simulink model "sim_linear_control_pos_v1"  (R2018a)
settings: Solver=ode3  StartTime=0.0  StopTime=t(end)  FixedStep=dt  RelTol=1e-3
values from neighbouring files (symbols this model uses):
  A = [-(Cf+Cr)/(m*Vx)  -(a*Cf-b*Cr)/(m*Vx)-Vx ... (first row only)    [lin_control_pos_v1.m]    (also in lin_control_y.m)
  B = [Cf/m; a*Cf/Iz]    [lin_control_pos_v1.m]    (also in lin_control_y.m)
  C = Col(3,:)    [lin_control_pos_v1.m]    (also in lin_control_y.m)
  CA = C*Aol    [lin_control_pos_v1.m]    (also in lin_control_y.m)
  invCB = pinv(C*Bol)    [lin_control_pos_v1.m]    (also in lin_control_y.m)
  K_ay = 8    [lin_control_pos_v1.m]    (also in lin_control_y.m = 4)
  K_chi = 2    [lin_control_pos_v1.m]
  K_Vy = 4    [lin_control_pos_v1.m]
  rho = 1/R    (= 0.05)    [lin_control_pos_v1.m]    (also in lin_control_y.m)
  Vx = 10/3.6    (= 2.77777777778)    [lin_control_pos_v1.m]    (also in lin_control_y.m)
  w = 10    [lin_control_pos_v1.m]    (also in lin_control_y.m)
settings Model: Creator=E183308  LastModifiedBy=E183308

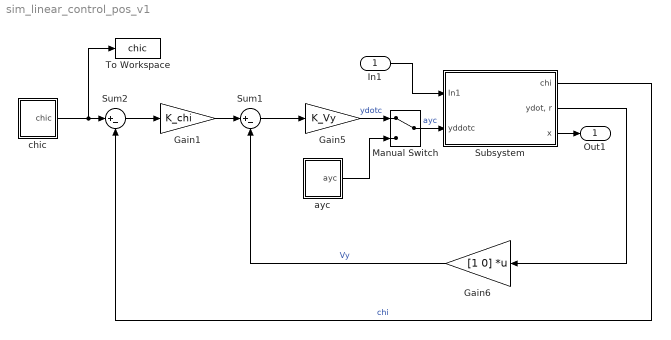
== system sim_linear_control_pos_v1 ==
  In1 : Inport
  Gain1 : Gain  Gain=K_chi
  Gain5 : Gain  Gain=K_Vy
  Gain6 : Gain  Gain=[1 0]  Multiplication=Matrix(K*u)
  Manual Switch : ManualSwitch
  Subsystem : Subsystem
  Sum1 : Sum  Inputs=|+-
  Sum2 : Sum  Inputs=|+-
  To Workspace : ToWorkspace  VariableName=chic  SampleTime=-1
  ayc : Subsystem
  chic : Subsystem
  Out1 : Outport
  wires:
  Gain5/1 -> Manual Switch/1  "ydotc"
  Sum1/1 -> Gain5/1
  Gain6/1 -> Sum1/2  "Vy"
  In1/1 -> Subsystem/1(In1)
  Manual Switch/1 -> Subsystem/2(yddotc)  "ayc"
  Subsystem/2("ydot, r") -> Gain6/1
  Subsystem/3(x) -> Out1/1
  Gain1/1 -> Sum1/1
  ayc/1(ayc) -> Manual Switch/2
  Subsystem/1(chi) -> Sum2/2  "chi"
  Sum2/1 -> Gain1/1
  chic/1(chic) -> To Workspace/1, Sum2/1

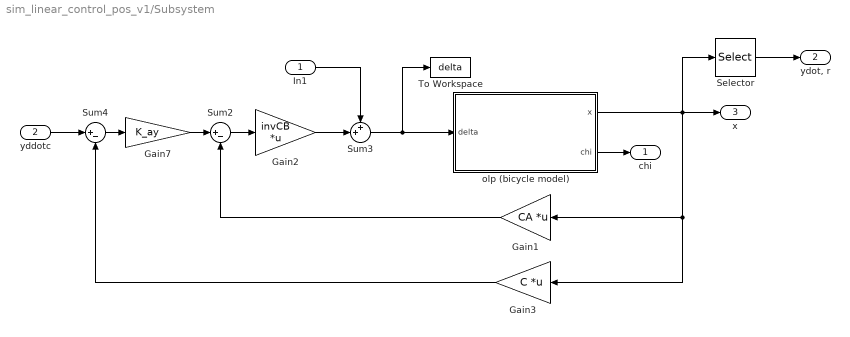
== system sim_linear_control_pos_v1/Subsystem ==
  In1 : Inport
  yddotc : Inport  Port=2
  Gain1 : Gain  Gain=CA  Multiplication=Matrix(K*u)
  Gain2 : Gain  Gain=invCB  Multiplication=Matrix(K*u)
  Gain3 : Gain  Gain=C  Multiplication=Matrix(K*u)
  Gain7 : Gain  Gain=K_ay
  Selector : Selector  InputPortWidth=5  IndexOptions=Index vector (dialog)  Indices=[1 2]  OutputSizes=1
  Sum2 : Sum  Inputs=|+-
  Sum3 : Sum  Inputs=++|
  Sum4 : Sum  Inputs=|+-
  To Workspace : ToWorkspace  VariableName=delta  SampleTime=-1
  olp (bicycle model) : Subsystem
  chi : Outport
  "ydot, r" : Outport  Port=2
  x : Outport  Port=3
  wires:
  yddotc/1 -> Sum4/1
  Gain3/1 -> Sum4/2
  Sum2/1 -> Gain2/1
  Sum4/1 -> Gain7/1
  Gain1/1 -> Sum2/2
  Gain7/1 -> Sum2/1
  olp (bicycle model)/1(x) -> Gain3/1, Gain1/1, x/1, Selector/1
  Selector/1 -> "ydot, r"/1
  Gain2/1 -> Sum3/2
  Sum3/1 -> To Workspace/1, olp (bicycle model)/1(delta)
  In1/1 -> Sum3/1
  olp (bicycle model)/2(chi) -> chi/1

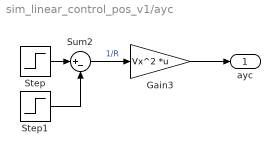
== system sim_linear_control_pos_v1/ayc ==
  Gain3 : Gain  Gain=Vx^2  Multiplication=Matrix(K*u)
  Step : Step  After=rho  SampleTime=0
  Step1 : Step  Time=5  After=rho  SampleTime=0
  Sum2 : Sum  Inputs=|+-
  ayc : Outport
  wires:
  Step1/1 -> Sum2/2
  Step/1 -> Sum2/1
  Sum2/1 -> Gain3/1  "1/R"
  Gain3/1 -> ayc/1

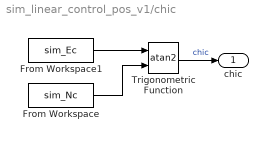
== system sim_linear_control_pos_v1/chic ==
  From Workspace : FromWorkspace  VariableName=sim_Nc  SampleTime=0
  From Workspace1 : FromWorkspace  VariableName=sim_Ec  SampleTime=0
  Trigonometric Function : Trigonometry  Operator=atan2
  chic : Outport
  wires:
  From Workspace1/1 -> Trigonometric Function/1
  From Workspace/1 -> Trigonometric Function/2
  Trigonometric Function/1 -> chic/1  "chic"

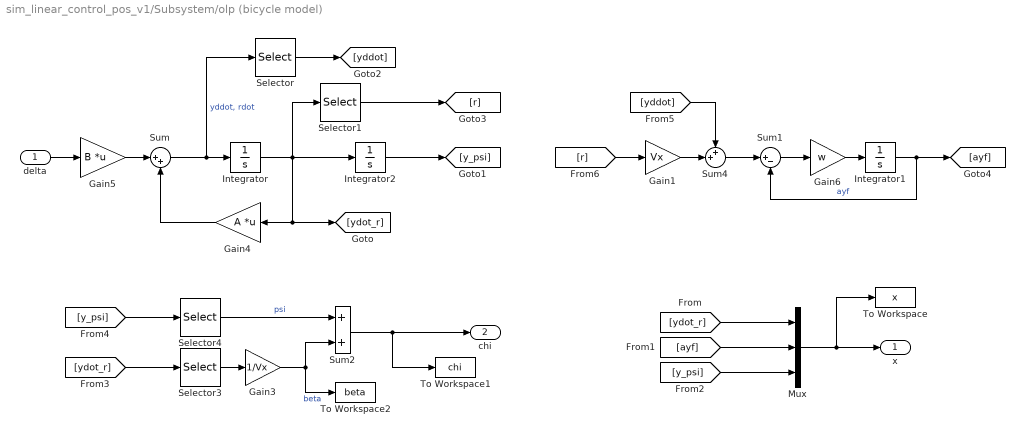
== system sim_linear_control_pos_v1/Subsystem/olp (bicycle model) ==
  delta : Inport
  Gain1 : Gain  Gain=Vx
  Gain3 : Gain  Gain=1/Vx
  Gain4 : Gain  Gain=A  Multiplication=Matrix(K*u)
  Gain5 : Gain  Gain=B  Multiplication=Matrix(K*u)
  Gain6 : Gain  Gain=w
  Integrator : Integrator  InitialCondition=[0;0]
  Integrator1 : Integrator
  Integrator2 : Integrator  InitialCondition=[0;0]
  Mux : Mux  Inputs=3
  Selector : Selector  InputPortWidth=2  IndexOptions=Index vector (dialog)  Indices=1  OutputSizes=1
  Selector1 : Selector  InputPortWidth=2  IndexOptions=Index vector (dialog)  Indices=2  OutputSizes=1
  Selector3 : Selector  InputPortWidth=2  IndexOptions=Index vector (dialog)  Indices=1  OutputSizes=1
  Selector4 : Selector  InputPortWidth=2  IndexOptions=Index vector (dialog)  Indices=2  OutputSizes=1
  Sum : Sum  Inputs=|++
  Sum1 : Sum  Inputs=|+-
  Sum2 : Sum
  Sum4 : Sum  Inputs=++|
  To Workspace : ToWorkspace  VariableName=x  SampleTime=-1
  To Workspace1 : ToWorkspace  VariableName=chi  SampleTime=-1
  To Workspace2 : ToWorkspace  VariableName=beta  SampleTime=-1
  x : Outport
  chi : Outport  Port=2
  wires:
  Integrator/1 -> Selector1/1, Integrator2/1, [ydot_r], Gain4/1
  delta/1 -> Gain5/1
  Gain5/1 -> Sum/1
  Gain4/1 -> Sum/2
  Gain6/1 -> Integrator1/1
  Sum1/1 -> Gain6/1
  Mux/1 -> x/1, To Workspace/1
  Integrator1/1 -> [ayf], Sum1/2  "ayf"
  Sum/1 -> Selector/1, Integrator/1  "yddot, rdot"
  Gain1/1 -> Sum4/2
  Sum4/1 -> Sum1/1
  Selector3/1 -> Gain3/1
  Selector4/1 -> Sum2/1  "psi"
  Gain3/1 -> To Workspace2/1, Sum2/2  "beta"
  Sum2/1 -> To Workspace1/1, chi/1
  [ydot_r] -> Mux/1
  [ayf] -> Mux/2
  [y_psi] -> Mux/3
  [ydot_r] -> Selector3/1
  [y_psi] -> Selector4/1
  Integrator2/1 -> [y_psi]
  Selector/1 -> [yddot]
  [yddot] -> Sum4/1
  Selector1/1 -> [r]
  [r] -> Gain1/1
